simulink model "blockdemo"  (Simulink 6.3)
settings: Solver=FixedStepDiscrete  StartTime=0.0  StopTime=20  FixedStep=1  RelTol=1e-3
InitFcn:
  | %% DSPBuilder Start
  | alt_dspbuilder_update_model(bdroot)
  | %% DSPBuilder End
libraries: allblocks_alteradspbuilder2 x5
settings Model: Creator=cpurcell  LastModifiedBy=delphick
settings OptimizationCC: BlockReduction=off  BooleanDataType=off  InlineInvariantSignals=on
settings DebuggingCC: SolverPrmCheckMsg=none
settings HardwareCC: TargetUnknown=on

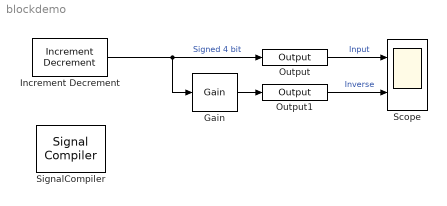
== system blockdemo ==
  Gain : allblocks_alteradspbuilder2/Gain  vgain=-20*pi/3  BusType=Signed Integer  bwl=8  bwr=0  pipeline=0  use_ena=off  use_aclr=off  lpm=off  MaskValue=1
  Increment Decrement : allblocks_alteradspbuilder2/Increment Decrement  BusType=Signed Integer  bwl=4  bwr=0  SpecifyClock=off  clr_value=0  direction=Increment  phase_selection=1  use_ena=off  use_sclr=off
  Output : allblocks_alteradspbuilder2/Output  iofile=C:\workspace_clean\Documentation\DesignExamples\Tutorials\UnitBlocks\Arithmetic\Gain\tb_blockdemo\blockdemo_Output.capture  BusType=Signed Integer  bwl=4  bwr=0  PORTTYPE=Output
  Output1 : allblocks_alteradspbuilder2/Output  iofile=C:\workspace_clean\Documentation\DesignExamples\Tutorials\UnitBlocks\Arithmetic\Gain\tb_blockdemo\blockdemo_Output1.capture  BusType=Signed Integer  bwl=10  bwr=0  PORTTYPE=Output
  Scope : Scope  NumInputPorts=2
      settings: TimeRange=20  YMin=-10~-200  YMax=10~200
  SignalCompiler : allblocks_alteradspbuilder2/Signal Compiler  DeviceFamily=Stratix IV  DeviceName=AUTO  EnableSignalTap=off  SignalTapDepth=128  UseBoardBlock=off  StpUseDefaultClock=on  StpClock=clock
  wires:
  Gain/1 -> Output1/1
  Increment Decrement/1 -> Gain/1, Output/1  "Signed 4 bit"
  Output/1 -> Scope/1  "Input"
  Output1/1 -> Scope/2  "Inverse"
